simulink model "simplebc_tl"  (Simulink 7.3)
settings: Solver=FixedStepDiscrete  SolverMode=SingleTasking  StartTime=0.0  StopTime=400  FixedStep=tsample  RelTol=1e-3
PreLoadFcn:
  | if exist('tl_preloadfcn','file'), tl_preloadfcn(gcs,101); end
PostLoadFcn:
  | if exist('tl_postloadfcn','file'), tl_postloadfcn(gcs,101); end
InitFcn:
  | if exist('tlds_init','file'), tlds_init(gcs); end
StartFcn:
  | if exist('tlds_start','file'), tlds_start(gcs); end
StopFcn:
  | if exist('tlds_stop','file'), tlds_stop(gcs); end
values from neighbouring files (symbols this model uses):
  fs_max = 4000    [simplebc_mdl.m]
  fs_min = 1000    [simplebc_mdl.m]
  maxcnt_heating = 10    [simplebc_mdl.m]
  maxcnt_ign = 3    [simplebc_mdl.m]
  maxcnt_preign = 2    [simplebc_mdl.m]
  maxcnt_prev1 = 3    [simplebc_mdl.m]
  maxcnt_prev2 = 8    [simplebc_mdl.m]
  maxcnt_standby = 10    [simplebc_mdl.m]
  srinp_resptime = 2    [simplebc_mdl.m]
  srinp_testcycletime = 3    [simplebc_mdl.m]
  sroutp_resptime = 2    [simplebc_mdl.m]
  sroutp_testcycletime = 3    [simplebc_mdl.m]
  tsample = 0.1    [simplebc_mdl.m]
libraries: tllib x6, simulink x6
(part 2 of 2)

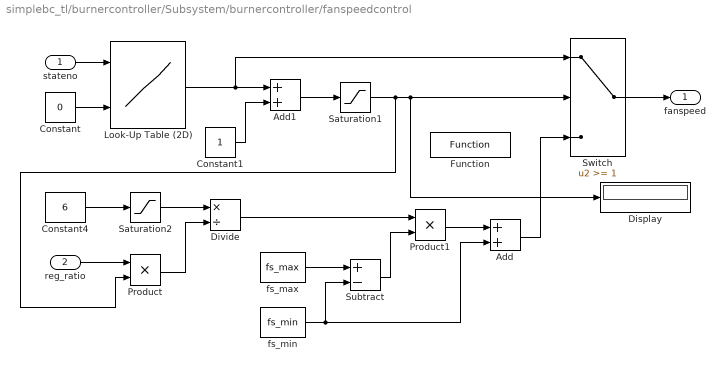
== system simplebc_tl/burnercontroller/Subsystem/burnercontroller/fanspeedcontrol ==
  stateno : Inport  OutDataType=sfix(16)  OutScaling=2^0
  reg_ratio : Inport  Port=2  OutDataType=sfix(16)  OutScaling=2^0
  Add : Sum  OutDataType=sfix(16)  OutScaling=2^-10  mask(TL_Sum){data={'logdata',{'plotchannels',[]},'output',{'type','UInt16','lsb',2^-2},'date',734178.39643339126}}
      settings: CopyFcn=set_param(gcb,'ReferenceBlock',''); set_param(gcb,'Tag','COPIED_DURING_UPGRADE');set_param(gcb,'CopyFcn','');  DeleteFcn=if exist('delete_tlblock','file')==2,delete_tlblock(gcbh);end  NameChangeFcn=if exist('rename_tlblock','file')==2,rename_tlblock(gcbh);end  OpenFcn=if exist('tl_open_blockdlg','file')==2,tl_open_blockdlg(gcbh);else,open_system(gcbh,'parameter');end
      mask Help: eval(['if exist(''tl_online_help'',''file'') == 2, tl_online_help(''Topic'',''TL_Sum''),else, web([''jar:file:///'',matlabroot,''/help/toolbox/simulink/help.jar!/slref/' lower(get_param(gcbh,'Blocktype')) '.html''], ''-helpbrowser''),end'])
      mask Display: plot([-0.05, 1.05, NaN, -0.05, 1.05],[.01, .01, NaN, .99, .99])
  Add1 : Sum  OutDataType=sfix(16)  OutScaling=2^-10  mask(TL_Sum){data={'logdata',{'plotchannels',[]},'output',{'type','UInt16'},'date',734178.39643303235}}
      settings: CopyFcn=set_param(gcb,'ReferenceBlock',''); set_param(gcb,'Tag','COPIED_DURING_UPGRADE');set_param(gcb,'CopyFcn','');  DeleteFcn=if exist('delete_tlblock','file')==2,delete_tlblock(gcbh);end  NameChangeFcn=if exist('rename_tlblock','file')==2,rename_tlblock(gcbh);end  OpenFcn=if exist('tl_open_blockdlg','file')==2,tl_open_blockdlg(gcbh);else,open_system(gcbh,'parameter');end
      mask Help: eval(['if exist(''tl_online_help'',''file'') == 2, tl_online_help(''Topic'',''TL_Sum''),else, web([''jar:file:///'',matlabroot,''/help/toolbox/simulink/help.jar!/slref/' lower(get_param(gcbh,'Blocktype')) '.html''], ''-helpbrowser''),end'])
      mask Display: plot([-0.05, 1.05, NaN, -0.05, 1.05],[.01, .01, NaN, .99, .99])
  Constant : Constant  Value=0  OutDataType=sfix(16)  OutScaling=2^0  mask(TL_Constant){data={'date',734178.39643266203}}
      settings: CopyFcn=set_param(gcb,'ReferenceBlock',''); set_param(gcb,'Tag','COPIED_DURING_UPGRADE');set_param(gcb,'CopyFcn','');  DeleteFcn=if exist('delete_tlblock','file')==2,delete_tlblock(gcbh);end  NameChangeFcn=if exist('rename_tlblock','file')==2,rename_tlblock(gcbh);end  OpenFcn=if exist('tl_open_blockdlg','file')==2,tl_open_blockdlg(gcbh);else,open_system(gcbh,'parameter');end
      mask Help: eval(['if exist(''tl_online_help'',''file'') == 2, tl_online_help(''Topic'',''TL_Constant''),else, web([''jar:file:///'',matlabroot,''/help/toolbox/simulink/help.jar!/slref/' lower(get_param(gcbh,'Blocktype')) '.html''], ''-helpbrowser''),end'])
      mask Display: plot([-0.05, 1.05, NaN, -0.05, 1.05],[.01, .01, NaN, .99, .99])
  Constant1 : Constant  OutDataType=sfix(16)  OutScaling=2^0  mask(TL_Constant){data={'date',734178.39643248846}}
      settings: CopyFcn=set_param(gcb,'ReferenceBlock',''); set_param(gcb,'Tag','COPIED_DURING_UPGRADE');set_param(gcb,'CopyFcn','');  DeleteFcn=if exist('delete_tlblock','file')==2,delete_tlblock(gcbh);end  NameChangeFcn=if exist('rename_tlblock','file')==2,rename_tlblock(gcbh);end  OpenFcn=if exist('tl_open_blockdlg','file')==2,tl_open_blockdlg(gcbh);else,open_system(gcbh,'parameter');end
      mask Help: eval(['if exist(''tl_online_help'',''file'') == 2, tl_online_help(''Topic'',''TL_Constant''),else, web([''jar:file:///'',matlabroot,''/help/toolbox/simulink/help.jar!/slref/' lower(get_param(gcbh,'Blocktype')) '.html''], ''-helpbrowser''),end'])
      mask Display: plot([-0.05, 1.05, NaN, -0.05, 1.05],[.01, .01, NaN, .99, .99])
  Constant4 : Constant  Value=6  OutDataType=sfix(16)  OutScaling=2^0  mask(TL_Constant){data={'date',734178.39643212967}}
      settings: CopyFcn=set_param(gcb,'ReferenceBlock',''); set_param(gcb,'Tag','COPIED_DURING_UPGRADE');set_param(gcb,'CopyFcn','');  DeleteFcn=if exist('delete_tlblock','file')==2,delete_tlblock(gcbh);end  NameChangeFcn=if exist('rename_tlblock','file')==2,rename_tlblock(gcbh);end  OpenFcn=if exist('tl_open_blockdlg','file')==2,tl_open_blockdlg(gcbh);else,open_system(gcbh,'parameter');end
      mask Help: eval(['if exist(''tl_online_help'',''file'') == 2, tl_online_help(''Topic'',''TL_Constant''),else, web([''jar:file:///'',matlabroot,''/help/toolbox/simulink/help.jar!/slref/' lower(get_param(gcbh,'Blocktype')) '.html''], ''-helpbrowser''),end'])
      mask Display: plot([-0.05, 1.05, NaN, -0.05, 1.05],[.01, .01, NaN, .99, .99])
  Display : Display
  Divide : Product  Inputs=*/  OutDataType=sfix(16)  OutScaling=2^-10  mask(TL_Product){data={'logdata',{'plotchannels',[]},'output',{'type','UInt16','lsb',2^-2},'date',734178.39643175923}}
      settings: CopyFcn=set_param(gcb,'ReferenceBlock',''); set_param(gcb,'Tag','COPIED_DURING_UPGRADE');set_param(gcb,'CopyFcn','');  DeleteFcn=if exist('delete_tlblock','file')==2,delete_tlblock(gcbh);end  NameChangeFcn=if exist('rename_tlblock','file')==2,rename_tlblock(gcbh);end  OpenFcn=if exist('tl_open_blockdlg','file')==2,tl_open_blockdlg(gcbh);else,open_system(gcbh,'parameter');end
      mask Help: eval(['if exist(''tl_online_help'',''file'') == 2, tl_online_help(''Topic'',''TL_Product''),else, web([''jar:file:///'',matlabroot,''/help/toolbox/simulink/help.jar!/slref/' lower(get_param(gcbh,'Blocktype')) '.html''], ''-helpbrowser''),end'])
      mask Display: plot([-0.05, 1.05, NaN, -0.05, 1.05],[.01, .01, NaN, .99, .99])
  Function : tllib/Function  SystemSampleTime=-1  data={'date',734178.39642018522}
  Look-Up Table (2D) : Lookup2D  RowIndex=[0 1 2 3 4 5 7 99]  Table=[0 0; 4000 4000; 4000 4000; 4000 4000; 3000 3000; 3000 3000; -1 -1; 0 0;]  LookUpMeth=Use Input Nearest  OutDataType=sfix(16)  OutScaling=2^0  SaturateOnIntegerOverflow=on  mask(TL_Lookup2D){data={'logdata',{'plotchannels',[]},'row',{'type','Int16'},'col',{'type','Int16'},'table',{'type','Int16','lsb',2^-2},'date',734178.39643121522}}
      settings: CopyFcn=set_param(gcb,'ReferenceBlock',''); set_param(gcb,'Tag','COPIED_DURING_UPGRADE');set_param(gcb,'CopyFcn','');  DeleteFcn=if exist('delete_tlblock','file')==2,delete_tlblock(gcbh);end  NameChangeFcn=if exist('rename_tlblock','file')==2,rename_tlblock(gcbh);end  OpenFcn=if exist('tl_open_blockdlg','file')==2,tl_open_blockdlg(gcbh);else,open_system(gcbh,'parameter');end
      mask Help: eval(['if exist(''tl_online_help'',''file'') == 2, tl_online_help(''Topic'',''TL_Lookup2D''),else, web([''jar:file:///'',matlabroot,''/help/toolbox/simulink/help.jar!/slref/' lower(get_param(gcbh,'Blocktype')) '.html''], ''-helpbrowser''),end'])
      mask Display: plot([-0.05, 1.05, NaN, -0.05, 1.05],[.01, .01, NaN, .99, .99])
  Product : Product  OutDataType=sfix(16)  OutScaling=2^0  RndMeth=Zero  mask(TL_Product){data={'logdata',{'plotchannels',[]},'output',{'type','UInt16','lsb',2^-2},'date',734178.39643031254}}
      settings: CopyFcn=set_param(gcb,'ReferenceBlock',''); set_param(gcb,'Tag','COPIED_DURING_UPGRADE');set_param(gcb,'CopyFcn','');  DeleteFcn=if exist('delete_tlblock','file')==2,delete_tlblock(gcbh);end  NameChangeFcn=if exist('rename_tlblock','file')==2,rename_tlblock(gcbh);end  OpenFcn=if exist('tl_open_blockdlg','file')==2,tl_open_blockdlg(gcbh);else,open_system(gcbh,'parameter');end
      mask Help: eval(['if exist(''tl_online_help'',''file'') == 2, tl_online_help(''Topic'',''TL_Product''),else, web([''jar:file:///'',matlabroot,''/help/toolbox/simulink/help.jar!/slref/' lower(get_param(gcbh,'Blocktype')) '.html''], ''-helpbrowser''),end'])
      mask Display: plot([-0.05, 1.05, NaN, -0.05, 1.05],[.01, .01, NaN, .99, .99])
  Product1 : Product  OutDataType=sfix(16)  OutScaling=2^0  RndMeth=Zero  mask(TL_Product){data={'logdata',{'plotchannels',[]},'output',{'type','UInt16','lsb',2^-2},'date',734178.39642995375}}
      settings: CopyFcn=set_param(gcb,'ReferenceBlock',''); set_param(gcb,'Tag','COPIED_DURING_UPGRADE');set_param(gcb,'CopyFcn','');  DeleteFcn=if exist('delete_tlblock','file')==2,delete_tlblock(gcbh);end  NameChangeFcn=if exist('rename_tlblock','file')==2,rename_tlblock(gcbh);end  OpenFcn=if exist('tl_open_blockdlg','file')==2,tl_open_blockdlg(gcbh);else,open_system(gcbh,'parameter');end
      mask Help: eval(['if exist(''tl_online_help'',''file'') == 2, tl_online_help(''Topic'',''TL_Product''),else, web([''jar:file:///'',matlabroot,''/help/toolbox/simulink/help.jar!/slref/' lower(get_param(gcbh,'Blocktype')) '.html''], ''-helpbrowser''),end'])
      mask Display: plot([-0.05, 1.05, NaN, -0.05, 1.05],[.01, .01, NaN, .99, .99])
  Saturation1 : Saturate  UpperLimit=1  LowerLimit=0  mask(TL_Saturate){data={'logdata',{'plotchannels',1},'output',{'type','UInt16','lsb',2^-2},'autoscaling',{'lowerheadroom',0},'date',734178.39642959496}}
      settings: CopyFcn=set_param(gcb,'ReferenceBlock',''); set_param(gcb,'Tag','COPIED_DURING_UPGRADE');set_param(gcb,'CopyFcn','');  DeleteFcn=if exist('delete_tlblock','file')==2,delete_tlblock(gcbh);end  NameChangeFcn=if exist('rename_tlblock','file')==2,rename_tlblock(gcbh);end  OpenFcn=if exist('tl_open_blockdlg','file')==2,tl_open_blockdlg(gcbh);else,open_system(gcbh,'parameter');end
      mask Help: eval(['if exist(''tl_online_help'',''file'') == 2, tl_online_help(''Topic'',''TL_Saturate''),else, web([''jar:file:///'',matlabroot,''/help/toolbox/simulink/help.jar!/slref/' lower(get_param(gcbh,'Blocktype')) '.html''], ''-helpbrowser''),end'])
      mask Display: plot([-0.05, 1.05, NaN, -0.05, 1.05],[.01, .01, NaN, .99, .99])
  Saturation2 : Saturate  UpperLimit=100  LowerLimit=0  mask(TL_Saturate){data={'logdata',{'plotchannels',[]},'date',734178.39642905095}}
      settings: CopyFcn=set_param(gcb,'ReferenceBlock',''); set_param(gcb,'Tag','COPIED_DURING_UPGRADE');set_param(gcb,'CopyFcn','');  DeleteFcn=if exist('delete_tlblock','file')==2,delete_tlblock(gcbh);end  NameChangeFcn=if exist('rename_tlblock','file')==2,rename_tlblock(gcbh);end  OpenFcn=if exist('tl_open_blockdlg','file')==2,tl_open_blockdlg(gcbh);else,open_system(gcbh,'parameter');end
      mask Help: eval(['if exist(''tl_online_help'',''file'') == 2, tl_online_help(''Topic'',''TL_Saturate''),else, web([''jar:file:///'',matlabroot,''/help/toolbox/simulink/help.jar!/slref/' lower(get_param(gcbh,'Blocktype')) '.html''], ''-helpbrowser''),end'])
      mask Display: plot([-0.05, 1.05, NaN, -0.05, 1.05],[.01, .01, NaN, .99, .99])
  Subtract : Sum  Inputs=+-  OutDataType=sfix(16)  OutScaling=2^-10  mask(TL_Sum){data={'logdata',{'plotchannels',[]},'date',734178.39642814815}}
      settings: CopyFcn=set_param(gcb,'ReferenceBlock',''); set_param(gcb,'Tag','COPIED_DURING_UPGRADE');set_param(gcb,'CopyFcn','');  DeleteFcn=if exist('delete_tlblock','file')==2,delete_tlblock(gcbh);end  NameChangeFcn=if exist('rename_tlblock','file')==2,rename_tlblock(gcbh);end  OpenFcn=if exist('tl_open_blockdlg','file')==2,tl_open_blockdlg(gcbh);else,open_system(gcbh,'parameter');end
      mask Help: eval(['if exist(''tl_online_help'',''file'') == 2, tl_online_help(''Topic'',''TL_Sum''),else, web([''jar:file:///'',matlabroot,''/help/toolbox/simulink/help.jar!/slref/' lower(get_param(gcbh,'Blocktype')) '.html''], ''-helpbrowser''),end'])
      mask Display: plot([-0.05, 1.05, NaN, -0.05, 1.05],[.01, .01, NaN, .99, .99])
  Switch : Switch  Threshold=1  mask(TL_Switch){data={'logdata',{'plotchannels',[]},'output',{'type','UInt16','lsb',2^-2},'threshold',{'scalar',1},'date',734178.39642778935}}
      settings: CopyFcn=set_param(gcb,'ReferenceBlock',''); set_param(gcb,'Tag','COPIED_DURING_UPGRADE');set_param(gcb,'CopyFcn','');  DeleteFcn=if exist('delete_tlblock','file')==2,delete_tlblock(gcbh);end  NameChangeFcn=if exist('rename_tlblock','file')==2,rename_tlblock(gcbh);end  OpenFcn=if exist('tl_open_blockdlg','file')==2,tl_open_blockdlg(gcbh);else,open_system(gcbh,'parameter');end
      mask Help: eval(['if exist(''tl_online_help'',''file'') == 2, tl_online_help(''Topic'',''TL_Switch''),else, web([''jar:file:///'',matlabroot,''/help/toolbox/simulink/help.jar!/slref/' lower(get_param(gcbh,'Blocktype')) '.html''], ''-helpbrowser''),end'])
      mask Display: plot([-0.05, 1.05, NaN, -0.05, 1.05],[.01, .01, NaN, .99, .99])
  fs_max : Constant  Value=fs_max  OutDataType=sfix(16)  OutScaling=2^0  mask(TL_Constant){data={'date',734178.39642724534}}
      settings: CopyFcn=set_param(gcb,'ReferenceBlock',''); set_param(gcb,'Tag','COPIED_DURING_UPGRADE');set_param(gcb,'CopyFcn','');  DeleteFcn=if exist('delete_tlblock','file')==2,delete_tlblock(gcbh);end  NameChangeFcn=if exist('rename_tlblock','file')==2,rename_tlblock(gcbh);end  OpenFcn=if exist('tl_open_blockdlg','file')==2,tl_open_blockdlg(gcbh);else,open_system(gcbh,'parameter');end
      mask Help: eval(['if exist(''tl_online_help'',''file'') == 2, tl_online_help(''Topic'',''TL_Constant''),else, web([''jar:file:///'',matlabroot,''/help/toolbox/simulink/help.jar!/slref/' lower(get_param(gcbh,'Blocktype')) '.html''], ''-helpbrowser''),end'])
      mask Display: plot([-0.05, 1.05, NaN, -0.05, 1.05],[.01, .01, NaN, .99, .99])
  fs_min : Constant  Value=fs_min  OutDataType=sfix(16)  OutScaling=2^0  mask(TL_Constant){data={'date',734178.39642687503}}
      settings: CopyFcn=set_param(gcb,'ReferenceBlock',''); set_param(gcb,'Tag','COPIED_DURING_UPGRADE');set_param(gcb,'CopyFcn','');  DeleteFcn=if exist('delete_tlblock','file')==2,delete_tlblock(gcbh);end  NameChangeFcn=if exist('rename_tlblock','file')==2,rename_tlblock(gcbh);end  OpenFcn=if exist('tl_open_blockdlg','file')==2,tl_open_blockdlg(gcbh);else,open_system(gcbh,'parameter');end
      mask Help: eval(['if exist(''tl_online_help'',''file'') == 2, tl_online_help(''Topic'',''TL_Constant''),else, web([''jar:file:///'',matlabroot,''/help/toolbox/simulink/help.jar!/slref/' lower(get_param(gcbh,'Blocktype')) '.html''], ''-helpbrowser''),end'])
      mask Display: plot([-0.05, 1.05, NaN, -0.05, 1.05],[.01, .01, NaN, .99, .99])
  fanspeed : Outport  OutDataType=sfix(16)  OutScaling=2^0
  wires:
  Add/1 -> Switch/3
  Constant1/1 -> Add1/2
  Look-Up Table (2D)/1 -> Switch/1, Add1/1
  Subtract/1 -> Product1/2
  fs_max/1 -> Subtract/1
  fs_min/1 -> Subtract/2, Add/2
  Product1/1 -> Add/1
  Divide/1 -> Product1/1
  Saturation2/1 -> Divide/1
  Product/1 -> Divide/2
  reg_ratio/1 -> Product/1
  Switch/1 -> fanspeed/1
  Saturation1/1 -> Product/2, Switch/2, Display/1
  Add1/1 -> Saturation1/1
  Constant/1 -> Look-Up Table (2D)/2
  stateno/1 -> Look-Up Table (2D)/1
  Constant4/1 -> Saturation2/1

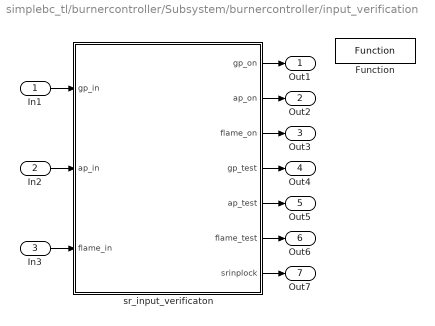
== system simplebc_tl/burnercontroller/Subsystem/burnercontroller/input_verification ==
  In1 : Inport  OutDataType=sfix(16)  OutScaling=2^0
  In2 : Inport  Port=2  OutDataType=sfix(16)  OutScaling=2^0
  In3 : Inport  Port=3  OutDataType=sfix(16)  OutScaling=2^0
  Function : tllib/Function  SystemSampleTime=-1  data={'date',734178.39641982643}
  sr_input_verificaton : Stateflow chart
  Out1 : Outport  OutDataType=sfix(16)  OutScaling=2^0
  Out2 : Outport  Port=2  OutDataType=sfix(16)  OutScaling=2^0
  Out3 : Outport  Port=3  OutDataType=sfix(16)  OutScaling=2^0
  Out4 : Outport  Port=4  OutDataType=sfix(16)  OutScaling=2^0
  Out5 : Outport  Port=5  OutDataType=sfix(16)  OutScaling=2^0
  Out6 : Outport  Port=6  OutDataType=sfix(16)  OutScaling=2^0
  Out7 : Outport  Port=7  OutDataType=sfix(16)  OutScaling=2^0
  wires:
  sr_input_verificaton/7(srinplock) -> Out7/1
  In3/1 -> sr_input_verificaton/3(flame_in)
  sr_input_verificaton/6(flame_test) -> Out6/1
  sr_input_verificaton/5(ap_test) -> Out5/1
  sr_input_verificaton/4(gp_test) -> Out4/1
  In2/1 -> sr_input_verificaton/2(ap_in)
  sr_input_verificaton/3(flame_on) -> Out3/1
  sr_input_verificaton/2(ap_on) -> Out2/1
  In1/1 -> sr_input_verificaton/1(gp_in)
  sr_input_verificaton/1(gp_on) -> Out1/1

== system simplebc_tl/burnercontroller/Subsystem/burnercontroller/lockcontroller ==
  mainctrlock : Inport  OutDataType=sfix(16)  OutScaling=2^0
  srinplock : Inport  Port=2  OutDataType=sfix(16)  OutScaling=2^0
  reset_in : Inport  Port=3  OutDataType=sfix(16)  OutScaling=2^0
  sroutplock : Inport  Port=4  OutDataType=sfix(16)  OutScaling=2^0
  lock_out_delay : UnitDelay  SampleTime=-1  mask(TL_UnitDelay){data={'logdata',{'plotchannels',[]},'output',{'type','Bool'},'state',{'type','Bool'},'date',734178.39642651624}}
      settings: CopyFcn=set_param(gcb,'ReferenceBlock',''); set_param(gcb,'Tag','COPIED_DURING_UPGRADE');set_param(gcb,'CopyFcn','');  DeleteFcn=if exist('delete_tlblock','file')==2,delete_tlblock(gcbh);end  NameChangeFcn=if exist('rename_tlblock','file')==2,rename_tlblock(gcbh);end  OpenFcn=if exist('tl_open_blockdlg','file')==2,tl_open_blockdlg(gcbh);else,open_system(gcbh,'parameter');end
      mask Help: eval(['if exist(''tl_online_help'',''file'') == 2, tl_online_help(''Topic'',''TL_UnitDelay''),else, web([''jar:file:///'',matlabroot,''/help/toolbox/simulink/help.jar!/slref/' lower(get_param(gcbh,'Blocktype')) '.html''], ''-helpbrowser''),end'])
      mask Display: plot([-0.05, 1.05, NaN, -0.05, 1.05],[.01, .01, NaN, .99, .99])
  lockctrl : Stateflow chart  TreatAsAtomicUnit=on
  unlock_out_delay : UnitDelay  SampleTime=-1  mask(TL_UnitDelay){data={'logdata',{'plotchannels',[]},'output',{'type','Bool'},'state',{'type','Bool'},'date',734178.39642597223}}
      settings: CopyFcn=set_param(gcb,'ReferenceBlock',''); set_param(gcb,'Tag','COPIED_DURING_UPGRADE');set_param(gcb,'CopyFcn','');  DeleteFcn=if exist('delete_tlblock','file')==2,delete_tlblock(gcbh);end  NameChangeFcn=if exist('rename_tlblock','file')==2,rename_tlblock(gcbh);end  OpenFcn=if exist('tl_open_blockdlg','file')==2,tl_open_blockdlg(gcbh);else,open_system(gcbh,'parameter');end
      mask Help: eval(['if exist(''tl_online_help'',''file'') == 2, tl_online_help(''Topic'',''TL_UnitDelay''),else, web([''jar:file:///'',matlabroot,''/help/toolbox/simulink/help.jar!/slref/' lower(get_param(gcbh,'Blocktype')) '.html''], ''-helpbrowser''),end'])
      mask Display: plot([-0.05, 1.05, NaN, -0.05, 1.05],[.01, .01, NaN, .99, .99])
  lock : Outport  OutDataType=sfix(16)  OutScaling=2^0
  unlock : Outport  Port=2  OutDataType=sfix(16)  OutScaling=2^0
  wires:
  srinplock/1 -> lockctrl/2(inplock)
  mainctrlock/1 -> lockctrl/3(mainctrlock)
  sroutplock/1 -> lockctrl/4(outplock)
  reset_in/1 -> lockctrl/1(reset_in)
  lockctrl/1(lock_out) -> lock_out_delay/1
  lock_out_delay/1 -> lock/1
  lockctrl/2(unlock_out) -> unlock_out_delay/1
  unlock_out_delay/1 -> unlock/1

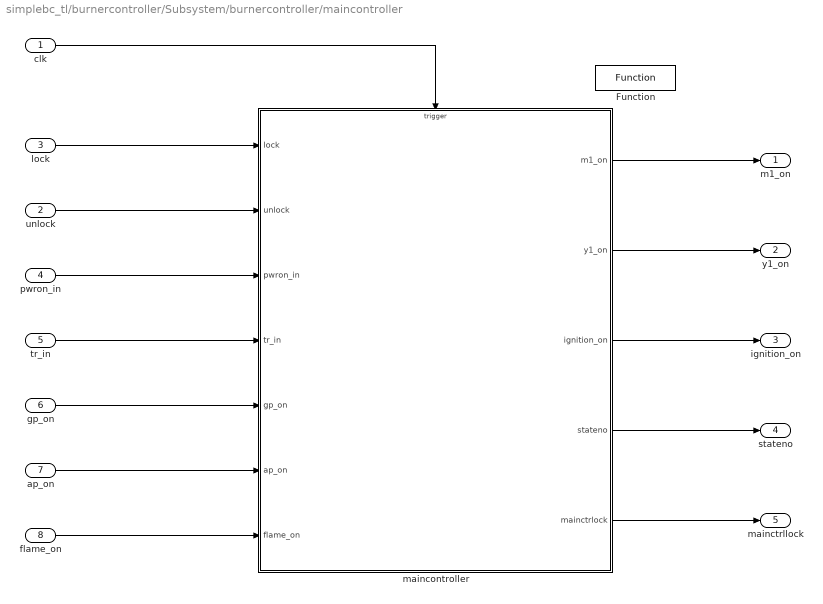
== system simplebc_tl/burnercontroller/Subsystem/burnercontroller/maincontroller ==
  clk : Inport  OutDataType=sfix(16)  OutScaling=2^0
  unlock : Inport  Port=2  OutDataType=sfix(16)  OutScaling=2^0
  lock : Inport  Port=3  OutDataType=sfix(16)  OutScaling=2^0
  pwron_in : Inport  Port=4  OutDataType=sfix(16)  OutScaling=2^0
  tr_in : Inport  Port=5  OutDataType=sfix(16)  OutScaling=2^0
  gp_on : Inport  Port=6  OutDataType=sfix(16)  OutScaling=2^0
  ap_on : Inport  Port=7  OutDataType=sfix(16)  OutScaling=2^0
  flame_on : Inport  Port=8  OutDataType=sfix(16)  OutScaling=2^0
  Function : tllib/Function  SystemSampleTime=-1  data={'date',734178.39641928242}
  maincontroller : Stateflow chart  TreatAsAtomicUnit=on
  m1_on : Outport  OutDataType=sfix(16)  OutScaling=2^0
  y1_on : Outport  Port=2  OutDataType=sfix(16)  OutScaling=2^0
  ignition_on : Outport  Port=3  OutDataType=sfix(16)  OutScaling=2^0
  stateno : Outport  Port=4  OutDataType=sfix(16)  OutScaling=2^0
  mainctrllock : Outport  Port=5  OutDataType=sfix(16)  OutScaling=2^0
  wires:
  clk/1 -> maincontroller/Trigger
  unlock/1 -> maincontroller/2(unlock)
  lock/1 -> maincontroller/1(lock)
  maincontroller/1(m1_on) -> m1_on/1
  pwron_in/1 -> maincontroller/3(pwron_in)
  maincontroller/2(y1_on) -> y1_on/1
  tr_in/1 -> maincontroller/4(tr_in)
  gp_on/1 -> maincontroller/5(gp_on)
  maincontroller/3(ignition_on) -> ignition_on/1
  ap_on/1 -> maincontroller/6(ap_on)
  maincontroller/4(stateno) -> stateno/1
  maincontroller/5(mainctrlock) -> mainctrllock/1
  flame_on/1 -> maincontroller/7(flame_on)

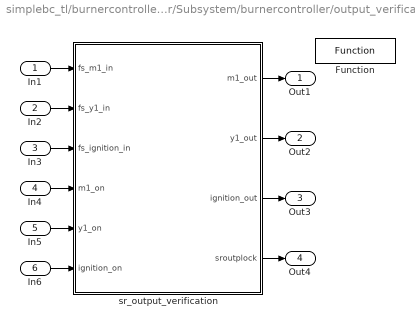
== system simplebc_tl/burnercontroller/Subsystem/burnercontroller/output_verification ==
  In1 : Inport  OutDataType=sfix(16)  OutScaling=2^0
  In2 : Inport  Port=2  OutDataType=sfix(16)  OutScaling=2^0
  In3 : Inport  Port=3  OutDataType=sfix(16)  OutScaling=2^0
  In4 : Inport  Port=4  OutDataType=sfix(16)  OutScaling=2^0
  In5 : Inport  Port=5  OutDataType=sfix(16)  OutScaling=2^0
  In6 : Inport  Port=6  OutDataType=sfix(16)  OutScaling=2^0
  Function : tllib/Function  SystemSampleTime=-1  data={'date',734178.3964181944}
  sr_output_verification : Stateflow chart
  Out1 : Outport  OutDataType=sfix(16)  OutScaling=2^0
  Out2 : Outport  Port=2  OutDataType=sfix(16)  OutScaling=2^0
  Out3 : Outport  Port=3  OutDataType=sfix(16)  OutScaling=2^0
  Out4 : Outport  Port=4  OutDataType=sfix(16)  OutScaling=2^0
  wires:
  In6/1 -> sr_output_verification/6(ignition_on)
  sr_output_verification/4(sroutplock) -> Out4/1
  In5/1 -> sr_output_verification/5(y1_on)
  sr_output_verification/3(ignition_out) -> Out3/1
  In4/1 -> sr_output_verification/4(m1_on)
  In3/1 -> sr_output_verification/3(fs_ignition_in)
  sr_output_verification/2(y1_out) -> Out2/1
  In2/1 -> sr_output_verification/2(fs_y1_in)
  sr_output_verification/1(m1_out) -> Out1/1
  In1/1 -> sr_output_verification/1(fs_m1_in)

== stateflow chart burnercontroller/Subsystem/burnercontroller/input_verification/sr_input_verificaton ==
  settings: sampleTime=0.05
  state gp_verification [parallel]
    settings: executionOrder=1
    state gpoff
      entry:
      gp_on=0;
      gp_test=0;
    state gpon
    state gptest
      entry: gp_test=1;
      exit: gp_test=0;
    (default) -> gpoff
    gpoff -> gpon : [gp_in]/gp_on=1;
    gpon -> gpoff [order 2] : after(srinp_resptime,tick)[!gp_in]/
        | gp_on=0;
    gpon -> gptest [order 1] : after(srinp_testcycletime,tick)
    gptest -> gpon [order 2] : after(srinp_resptime,tick)[!gp_in]
    gptest -> gpoff [order 1] : after(srinp_resptime,tick) [gp_in]/ srinplock=1;
  state ap_verification [parallel]
    settings: executionOrder=2
    state aptest
      entry: ap_test=1;
      exit: ap_test=0;
    state apoff
      entry:
      ap_on=0;
      ap_test=0;
    state apon
    (default) -> apoff
    apon -> aptest [order 1] : after(srinp_testcycletime,tick)
    apoff -> apon : [ap_in]/ap_on=1;
    aptest -> apon [order 2] : after(srinp_resptime,tick) [!ap_in]
    apon -> apoff [order 2] : after(srinp_resptime,tick)[! ap_in]/
        | ap_on=0;
    aptest -> apoff [order 1] : after(srinp_resptime,tick) [ap_in]/ srinplock=1;
  state flame_verification [parallel]
    settings: executionOrder=3
    state flameon
    state flameoff
      entry:
      flame_on=0;
      flame_test=0;
    state flametest
      entry: flame_test=1;
      exit: flame_test=0;
    (default) -> flameoff
    flameon -> flametest [order 1] : after(srinp_testcycletime,tick)
    flameoff -> flameon : [flame_in]/flame_on=1;
    flametest -> flameon [order 2] : after(srinp_resptime,tick) [!flame_in]
    flameon -> flameoff [order 2] : after(srinp_resptime,tick)[! flame_in]/
        | flame_on=0;
    flametest -> flameoff [order 1] : after(srinp_resptime,tick) [flame_in]/ srinplock=1;
  data: gp_in input boolean; ap_in input boolean; flame_in input boolean; gp_on output boolean =0; ap_on output boolean =0; flame_on output boolean =0; gp_test output boolean =0; ap_test output boolean =0; flame_test output boolean =0; srinplock output boolean =0; srinp_testcycletime parameter uint8 =10; srinp_resptime parameter uint8 =3
  data gp_in settings: description=$TL$ type=Bool; createinputvariable=1; $TL$
  data ap_in settings: description=$TL$ type=Bool; createinputvariable=1; $TL$
  data flame_in settings: description=$TL$ type=Bool; createinputvariable=1; $TL$
  data gp_on settings: description=$TL$ type=Bool; $TL$
  data ap_on settings: description=$TL$ type=Bool; $TL$
  data flame_on settings: description=$TL$ type=Bool; $TL$
  data gp_test settings: description=$TL$ type=Bool; $TL$
  data ap_test settings: description=$TL$ type=Bool; $TL$
  data flame_test settings: description=$TL$ type=Bool; $TL$
  data srinplock settings: description=$TL$ type=Bool; $TL$
  data srinp_testcycletime settings: description=$TL$ type=UInt8; class=CAL; $TL$
  data srinp_resptime settings: description=$TL$ type=UInt8; class=CAL; $TL$

== stateflow chart burnercontroller/Subsystem/burnercontroller/lockcontroller/lockctrl ==
  state unlocked
  state locked
    entry:
    lock_out=1;
    unlock_out=0;
  state unlocking
  unlocked -> locked : [inplock || mainctrlock || outplock]
  (default) -> unlocked
  locked -> unlocking : [reset_in]/rescnt=0;
  unlocking -> unlocked [order 2] : [!reset_in && rescnt >15 && rescnt < 60]/unlock_out=1;lock_out=0;
  unlocking -> locked [order 3] : [!reset_in &&  (rescnt <16 || rescnt > 59)]
  unlocking -> unlocking [order 1] : [reset_in && rescnt < 65]/rescnt++;
  data: lock_out output boolean =0; unlock_out output boolean =0; reset_in input boolean; rescnt local uint8 [0..65] =0; inplock input boolean; mainctrlock input boolean; outplock input boolean
  data lock_out settings: description=$TL$ type=Bool; $TL$
  data unlock_out settings: description=$TL$ type=Bool; $TL$
  data reset_in settings: description=$TL$ type=Bool; createinputvariable=1; $TL$
  data rescnt settings: description=$TL$ type=UInt8; $TL$
  data inplock settings: description=$TL$ type=Bool; createinputvariable=1; $TL$
  data mainctrlock settings: description=$TL$ type=Bool; createinputvariable=1; $TL$
  data outplock settings: description=$TL$ type=Bool; createinputvariable=1; $TL$

== stateflow chart burnercontroller/Subsystem/burnercontroller/maincontroller/maincontroller ==
  state systemcheck
    entry:
    m1_on=0;
    y1_on=0;
    ignition_on=0;
    stateno=0;
  state blocking
    entry:
    m1_on=0;
    y1_on=0;
    ignition_on=0;
    stateno=99;
    mainctrlock=1;
  state preventilation1
    entry: stateno=2;
  state standby
    entry: m1_on=0;y1_on=0;ignition_on=0;stateno=1;
  state heating
    entry: stateno=7;
  state preventilation2
    entry: stateno=3;
  state ignition
    entry: stateno=5;
  state preignition
    entry: stateno=4;
  standby -> systemcheck [order 1] : after(maxcnt_standby,clk)
  systemcheck -> standby [order 1] : after(2,clk)[pwron_in > 186]
  standby -> preventilation1 [order 2] : [tr_in && !lock]
      | /m1_on=1;
  (junction 73) -> standby
  preventilation1 -> (junction 73) [order 2] : [!tr_in]
  preventilation2 -> (junction 73) [order 2] : [!tr_in]
  heating -> (junction 73) [order 5] : [!tr_in]
  preventilation1 -> preventilation2 [order 1] : after(maxcnt_prev1,clk)[gp_on && !lock]
  blocking -> systemcheck : [unlock]/
      | mainctrlock=0;
  preventilation2 -> preignition [order 1] : after(maxcnt_prev2,clk)[gp_on && ap_on && !lock]
      | /ignition_on=1;
  preignition -> ignition [order 1] : after(maxcnt_preign,clk)[gp_on && ap_on ...
      | && !flame_on && !lock]/y1_on=1;
  ignition -> heating [order 1] : after(maxcnt_ign,clk)[gp_on && ap_on ...
      | && flame_on && !lock]/ignition_on=0;
  heating -> systemcheck [order 1] : after(maxcnt_heating,clk)
  systemcheck -> blocking [order 2] : [lock]
  standby -> blocking [order 3] : [lock]
  preventilation1 -> blocking [order 4] : [lock]
  preventilation1 -> blocking [order 3] : [!gp_on]
  preventilation2 -> blocking [order 4] : [lock]
  preventilation2 -> blocking [order 3] : [!gp_on || !ap_on]
  preignition -> blocking [order 3] : [lock]
  preignition -> blocking [order 2] : [!gp_on || !ap_on || flame_on]
  ignition -> blocking [order 3] : [lock || !gp_on || !ap_on]
  ignition -> blocking [order 2] : after(maxcnt_ign,clk)[!flame_on]
  heating -> blocking [order 4] : [!gp_on || !ap_on || !flame_on]
  heating -> blocking [order 3] : [lock]
  (default) -> systemcheck
  heating -> systemcheck [order 2] : [pwron_in<187]
  standby -> systemcheck [order 4] : [pwron_in < 187]
  data: lock input boolean; unlock input boolean; pwron_in input uint8 [0..253]; tr_in input boolean; gp_on input boolean; ap_on input boolean; flame_on input boolean; m1_on output boolean =0; y1_on output boolean =0; ignition_on output boolean =0; stateno output uint8 =0; mainctrlock output boolean =0; maxcnt_prev1 parameter uint8 =50; maxcnt_prev2 parameter uint8 =200; maxcnt_ign parameter uint8 =30; maxcnt_preign parameter uint8 =20; maxcnt_heating parameter uint8 =250; maxcnt_standby parameter uint8 =250
  data lock settings: description=$TL$ type=Bool; createinputvariable=1; $TL$
  data unlock settings: description=$TL$ type=Bool; createinputvariable=1; $TL$
  data pwron_in settings: description=$TL$ type=UInt8; createinputvariable=1; $TL$
  data tr_in settings: description=$TL$ type=Bool; createinputvariable=1; $TL$
  data gp_on settings: description=$TL$ type=Bool; createinputvariable=1; $TL$
  data ap_on settings: description=$TL$ type=Bool; createinputvariable=1; $TL$
  data flame_on settings: description=$TL$ type=Bool; createinputvariable=1; $TL$
  data m1_on settings: description=$TL$ type=Bool; $TL$
  data y1_on settings: description=$TL$ type=Bool; $TL$
  data ignition_on settings: description=$TL$ type=Bool; $TL$
  data stateno settings: description=$TL$ type=UInt8; $TL$
  data mainctrlock settings: description=$TL$ type=Bool; $TL$
  data maxcnt_prev1 settings: description=$TL$ type=UInt8; class=CAL; $TL$
  data maxcnt_prev2 settings: description=$TL$ type=UInt8; class=CAL; $TL$
  data maxcnt_ign settings: description=$TL$ type=UInt8; class=CAL; $TL$
  data maxcnt_preign settings: description=$TL$ type=UInt8; class=CAL; $TL$
  data maxcnt_heating settings: description=$TL$ type=UInt8; class=CAL; $TL$
  data maxcnt_standby settings: description=$TL$ type=UInt8; class=CAL; $TL$
  events: clk input RISING_EDGE_EVENT

== stateflow chart burnercontroller/Subsystem/burnercontroller/output_verification/sr_output_verification ==
  state y1_verification [parallel]
    settings: executionOrder=2
    state y1off
      entry:
      y1_out=0;
    state y1on
    state y1test
      entry: y1_out=0;
    y1test -> y1off [order 1] : after(sroutp_resptime,tick) [!fs_y1_in]/ sroutplock=1;
    y1test -> y1on [order 2] : after(sroutp_resptime,tick) [fs_y1_in]/
        | y1_out=1;
    (default) -> y1off
    y1on -> y1off [order 2] : [!y1_on]/y1_out=0;
    y1off -> y1on : [y1_on]/y1_out=1;
    y1on -> y1test [order 1] : after(sroutp_testcycletime,tick)
  state m1_verification [parallel]
    settings: executionOrder=1
    state m1on
    state m1off
      entry:
      m1_out=0;
    state m1test
      entry: m1_out=0;
    (default) -> m1off
    m1on -> m1test [order 1] : after(sroutp_testcycletime,tick)
    m1off -> m1on : [m1_on]/m1_out=1;
    m1on -> m1off [order 2] : [!m1_on]/m1_out=0;
    m1test -> m1on [order 2] : after(sroutp_resptime,tick) [fs_m1_in]/
        | m1_out=1;
    m1test -> m1off [order 1] : after(sroutp_resptime,tick) [!fs_m1_in]/ sroutplock=1;
  state ign_verification [parallel]
    settings: executionOrder=3
    state ignitionon
    state ignoff
      entry:
      ignition_out=0;
    state ignitiontest
      entry:
      ignition_out=0;
    (default) -> ignoff
    ignitionon -> ignitiontest [order 1] : after(sroutp_testcycletime,tick)
    ignoff -> ignitionon : [ignition_on]/ignition_out=1;
    ignitionon -> ignoff [order 2] : [!ignition_on]/ignition_out=0;
    ignitiontest -> ignitionon [order 2] : after(sroutp_resptime,tick) [fs_ignition_in]/
        | ignition_out=1;
    ignitiontest -> ignoff [order 1] : after(sroutp_resptime,tick) [!fs_ignition_in]/ sroutplock=1;
  data: fs_m1_in input boolean; fs_y1_in input boolean; fs_ignition_in input boolean; m1_out output boolean =0; m1_on input boolean; y1_on input boolean; ignition_on input boolean; y1_out output boolean =0; ignition_out output boolean =0; sroutplock output boolean =0; sroutp_testcycletime parameter uint8 =10; sroutp_resptime parameter uint8 =2
  data fs_m1_in settings: description=$TL$ type=Bool; createinputvariable=1; $TL$
  data fs_y1_in settings: description=$TL$ type=Bool; createinputvariable=1; $TL$
  data fs_ignition_in settings: description=$TL$ type=Bool; createinputvariable=1; $TL$
  data m1_out settings: description=$TL$ type=Bool; $TL$
  data m1_on settings: description=$TL$ type=Bool; createinputvariable=1; $TL$
  data y1_on settings: description=$TL$ type=Bool; createinputvariable=1; $TL$
  data ignition_on settings: description=$TL$ type=Bool; createinputvariable=1; $TL$
  data y1_out settings: description=$TL$ type=Bool; $TL$
  data ignition_out settings: description=$TL$ type=Bool; $TL$
  data sroutplock settings: description=$TL$ type=Bool; $TL$
  data sroutp_testcycletime settings: description=$TL$ type=UInt8; class=CAL; $TL$
  data sroutp_resptime settings: description=$TL$ type=UInt8; class=CAL; $TL$
